simulink library "Ampere_Library"  (R2022b)
settings: Solver=FixedStepDiscrete  StartTime=0  StopTime=10.0  RelTol=1e-3  EnableMultiTasking=on
undefined symbols (not defined in the file or in its folder): A_INST_double, Dem_EventStatusType, ECU_AMBIENT_TEMPERATURE, SET_ECU_AMBIENT_TEMPERATURE, SlDemoSign, Std_ReturnType
libraries: simulink x13
(part 2 of 10)

== system Ampere_Library/User_Defined_Libraries/Discontinuities ==
  note: Saturation and Crossing
  note: Min/Max and DeadZone
  note: Hysteresis and Relays
  note: Discontinuities
  A_DetectSaturation : Subsystem  Tag=[LIB]  mask(A_DetectSaturation){SATOnIntegerOverflow=off}
      mask prompts: SATOnIntegerOverflow "Saturate on integer overflow"
      mask help:
      | Limit input signal to the upper and lower saturation values. Saturation of the [2](input) by entry [1] (maximum) and entry [3] (minimum). Output (sat) will be any of the following values
      |   0 : Input is within the threshold range
      |   1 : Input is less than or equal to minimum threshold
      |   2 : Input is greater than or equal to maximum threshold
      |   3 : The minimum threshold is equal to the maximum threshold.
      |
      | Notes:
      | 1. Second output(sat) is always uint8 datatype.
      | 2. Second output (sat) will be 2
      | if upper saturation value is less than lower saturation value.
      | e.g., if upper is -10 and lower is 10 , then output sat will be 2.
      mask init:
      | %% Internal Parameters
      | SatPas = uint8(0);
      | Satmin = uint8(1);
      | SatMax = uint8(2);
      | UpEqLow = uint8(3);
      settings: AttributesFormatString=%<MaskType>
      mask TypeOptions SATOnIntegerOverflow: Max/SaturateOnIntegerOverflow | Min/SaturateOnIntegerOverflow
      mask Callback SATOnIntegerOverflow:
      | if strcmp(get_param(gcb,'SATOnIntegerOverflow'),'on')
      |     % Display the SaturateOnOverflow parameter
      |     set_param(gcb, 'AttributesFormatString', sprintf('%%<MaskType>\n SAT = on'));
      | else
      |     % Do not display the SaturateOnOverflow parameter
      |     set_param(gcb, 'AttributesFormatString', sprintf('%%<MaskType>\n'));
      | end
      mask Display:
      | %% Plot saturation and axes
      | plot([.8,.6,.4,.2],[.7,.7,.3,.3]);
      | plot([.5,.5],[0.25,.75]);
      | plot([.85,.15],[.5,.5]);
  A_HiThresHys_HighIncl : Subsystem  Tag=[LIB]  mask(A_HiThresHys_HighIncl){Sat_Required=off}
      mask prompts: Sat_Required "Saturate on integer overflow for sum block"
      mask help:
      | Hysteresis Function
      |
      | The block produces a flag that indicates
      | if the input (val) is within the Hysteresis phase
      | defined by hysw (Hysteresis width) and thrs (Threshold).
      |
      | Hys Type  :  Minus
      | Lower Threshold  :  Not Included
      | Upper Threshold  :  Included
      | Lower Hys Flag Value  :  0
      | Upper Hys Flag Value  :  1
      |
      | I/O
      | val     :  Value
      | thrs    :  Threshold Value
      | hysw  :  Hysteresis Width
      |
      | flag :  Answer Flag Value
      |
      | set   : val >= thrs
      | clear : val < thrs - hysw
      | hold  : thrs - hysw <= val < thrs (hold previous value)
      mask init:
      | %% Internal Parameter
      | Initial_condition = 0;
      settings: AttributesFormatString=%<MaskType>
      mask TypeOptions Sat_Required: Sum/SaturateOnIntegerOverflow
      mask Callback Sat_Required:
      | if strcmp(get_param(gcb,'Sat_Required'),'on')
      |     % Display the SaturateOnOverflow parameter
      |     set_param(gcb, 'AttributesFormatString',sprintf('%%<MaskType>\nSAT = on'));
      | else
      |     % Do not display the SaturateOnOverflow parameter
      |     set_param(gcb, 'AttributesFormatString',sprintf('%%<MaskType>\n'));
      | end
      mask Display:
      | %% Data to move up all objects
      | Moveup = .15;
      | 
      | %% Left to right arrow
      | plot([0.62 0.64 0.62], Moveup+[0.27 0.30 0.33]);
      | 
      | %% Right to left arrow
      | plot([0.41 0.39 0.41], Moveup+[0.73 0.70 0.67]);
      | 
      | %% Down up arrow
      | plot([0.62 0.64 0.66], Moveup+[0.66 0.68 0.66]);
      | 
      | %% Up down arrow
      | plot([0.4 0.38 0.36], Moveup+[0.34 0.32 0.34]);
      | 
      | %% Draw paths
      | plot([0.20 0.70], Moveup+[0.30 0.30]);
      | plot([0.64 0.64], Moveup+[0.30 0.70]);
      | plot([0.38 0.80], Moveup+[0.70 0.70]);
      | plot([0.38 0.38], Moveup+[0.30 0.70]);
      | 
      | %% Put texts
      | text(0.60, Moveup+0.15, '   x\n(thrs)');
      | text(0.22, Moveup+0.15, '         z \n(thrs - HysW)');
      | text(0.66, Moveup+0.5, 'val >= x\n   (set)');
      | text(0.41, Moveup+0.5, 'z<=val<x\n  (hold)');
      | text(0.20, Moveup+0.5, 'val < z\n   (clr)');
  A_HiThresHys_LowIncl : Subsystem  Tag=[LIB]  mask(A_HiThresHys_LowIncl){Sat_Required=off}
      mask prompts: Sat_Required "Saturate on integer overflow for Sum Block"
      mask help:
      | Hysteresis Function
      |
      | The block produces a flag that indicates
      | if the input (val) is within the Hysteresis phase
      | defined by hysw (Hysteresis width) and thrs (Threshold).
      |
      | Hys Type  :  Minus
      | Lower Threshold  :  Included
      | Upper Threshold  :  Not Included
      | Lower Hys Flag Value  :  0
      | Upper Hys Flag Value  :  1
      |
      | I/O
      | val     :  Value
      | thrs    :  Threshold Value
      | hysw  :  Hysteresis Width
      |
      | flag :  Answer Flag Value
      |
      | set   : val > thrs
      | clear : val <= thrs - hysw
      | hold  : thrs - hysw < val <= thrs (hold previous value)
      mask init:
      | %% Internal Parameter
      | Initial_condition = 0;
      settings: AttributesFormatString=%<MaskType>
      mask TypeOptions Sat_Required: Sum/SaturateOnIntegerOverflow
      mask Callback Sat_Required:
      | if strcmp(get_param(gcb,'Sat_Required'),'on')
      |     % Display the SaturateOnOverflow parameter
      |     set_param(gcb, 'AttributesFormatString',sprintf('%%<MaskType>\nSAT = on'));
      | else
      |     % Do not display the SaturateOnOverflow parameter
      |     set_param(gcb, 'AttributesFormatString',sprintf('%%<MaskType>\n'));
      | end
      mask Display:
      | %% Data to move up all objects
      | Moveup = .15;
      | 
      | %% Left to right arrow
      | plot([0.62 0.64 0.62], Moveup+[0.27 0.30 0.33]);
      | 
      | %% Right to left arrow
      | plot([0.41 0.39 0.41], Moveup+[0.73 0.70 0.67]);
      | 
      | %% Down up arrow
      | plot([0.62 0.64 0.66], Moveup+[0.66 0.68 0.66]);
      | 
      | %% Up down arrow
      | plot([0.4 0.38 0.36], Moveup+[0.34 0.32 0.34]);
      | 
      | %% Draw paths
      | plot([0.20 0.70], Moveup+[0.30 0.30]);
      | plot([0.64 0.64], Moveup+[0.30 0.70]);
      | plot([0.38 0.80], Moveup+[0.70 0.70]);
      | plot([0.38 0.38], Moveup+[0.30 0.70]);
      | 
      | %% Put texts
      | text(0.60, Moveup+0.15, '   x\n(thrs)');
      | text(0.22, Moveup+0.15, '         z \n(thrs - HysW)');
      | text(0.66, Moveup+0.5, 'val > x\n(set)')
      | text(0.41, Moveup+0.5, 'z<val<=x\n  (hold)')
      | text(0.18, Moveup+0.5, 'val <= z\n   (clr)')
  A_HitCrossing : Subsystem  Tag=[LIB]  mask(A_HitCrossing){offset=50, direction=either, tolerance=double tolerance - eps('double'), user_tol=1, Sat_Required=off}
      mask prompts: offset "Hit crossing offset:"; direction "Hit crossing direction"; tolerance "Tolerance for Offset"; user_tol "User Defined Tolerance"; Sat_Required "Saturate on integer overflow"
      mask help: Detects when the input signal 'U' reaches the Hit crossing offset parameter value in the direction specified by the Hit crossing direction parameter. If the input signal crosses the offset value in the specified direction, the block outputs 1 at the crossing time. If the input signal reaches the offset value in the specified direction and then remains at the offset value, the block outputs 'Out' 1 from the hit time till the time when signal leaves the offset value. If the input signal is constant and equal to the offset value, the block outputs 1 only if the direction is either. For variable-step solvers, Simulink takes a time step before and after the hit crossing time.
      mask init:
      | %% Internal Parameter
      | INI_VAL = 0;
      | 
      | %% Update internal blocks depending of the selected HitCrossing
      | switch direction
      |     case 1
      |         % case rising
      |         set_param([gcb '/VarFrom'],'GotoTag','rise_fall_out');
      |         set_param([gcb '/VarFrom1'],'GotoTag','false');
      |         set_param([gcb '/Var_RO1'],'Operator','>=');
      |         set_param([gcb '/Var_RO2'],'Operator','<');
      |         set_param([gcb '/Var_RO3'],'Operator','>');
      |         set_param([gcb '/Var_RO4'],'Operator','<=');
      |     case 2
      |         % case falling
      |         set_param([gcb '/VarFrom'],'GotoTag','rise_fall_out');
      |         set_param([gcb '/VarFrom1'],'GotoTag','false');
      |         set_param([gcb '/Var_RO1'],'Operator','<=');
      |         set_param([gcb '/Var_RO2'],'Operator','>');
      |         set_param([gcb '/Var_RO3'],'Operator','<');
      |         set_param([gcb '/Var_RO4'],'Operator','>=');
      |     case 3
      |         % case either
      |         set_param([gcb '/VarFrom'],'GotoTag','either');
      |         set_param([gcb '/VarFrom1'],'GotoTag','compare_out');
      | end
      | 
      | %% Compute Tolerance
      | switch tolerance
      |     case 1
      |         tol = eps('double');
      |     case 2
      |         tol = eps('single');
      |     case 3
      |         tol = 0;
      |     case 4
      |         tol = user_tol;
      | end
      | 
      | %% Create the infos to display below the block depending of the Mask Options
      | % Always display MaskType
      | Attrib = '%<MaskType>';
      | % Conditionnally adding Tolerance
      | if strcmp(get_param(gcb,'tolerance'),'User Defined')
      |     Attrib = [Attrib '\nTol = %<user_tol>'];
      | end
      | % Conditionnally adding Sat
      | if strcmp(get_param(gcb,'Sat_Required'),'on')
      |     Attrib = [Attrib '\nSAT = on'];
      | end
      | % Update the display
      | set_param(gcb,'AttributesFormatString',Attrib);
      settings: AttributesFormatString=%<MaskType>
      mask TypeOptions direction: rising | falling | either
      mask TypeOptions tolerance: double tolerance - eps('double') | single tolerance - eps('single') | Absolute Zero | User Defined
      mask Callback tolerance:
      | %% Make visible or not the Tolerance (update 2nd element of MaskVisibilities)
      | MaskVisibilities = get_param(gcb,'MaskVisibilities');
      | if strcmp(get_param(gcb,'tolerance'),'User Defined')
      |     MaskVisibilities{4} = 'on';
      | else
      |     MaskVisibilities{4} = 'off';
      | end
      | set_param(gcb,'MaskVisibilities',MaskVisibilities);
      mask TypeOptions Sat_Required: Add/SaturateOnIntegerOverflow | Add1/SaturateOnIntegerOverflow
      mask Display:
      | %% Plot horizontal and diagonal lines
      | plot([-1,1],[0,0]);
      | plot([-1,1],[-1,1]);
      | 
      | %% Plot the arrows depending of the mask option
      | if strcmp(get_param(gcb,'direction'),'either')
      |     plot([0,0],[-.5,.5]); % centre line
      |     plot([-.1,0],[.3,.5]); % upward arrow
      |     plot([0,.1],[.5,.3]); % upward arrow
      |     plot([0,.1],[-.5,-.3]) % down arrow
      |     plot([0,-.1],[-.5,-.3]) % down arrow
      | elseif strcmp(get_param(gcb,'direction'),'rising')
      |     plot([0,0],[0,.5]); % centre line
      |     plot([-.1,0],[.3,.5]); % upward line
      |     plot([0,.1],[.5,.3]); % upward arrow
      | elseif strcmp(get_param(gcb,'direction'),'falling')
      |     plot([0,0],[0,-.5]); % centre line
      |     plot([0,.1],[-.5,-.3]); % down arrow
      |     plot([0,-.1],[-.5,-.3]); % down arrow
      | end
      | 
      | %% Add the Offset value above as text
      | text(0,.85,sprintf('Offset = %s', get(gcbh,'offset')),'HorizontalAlignment','center')
  A_Hysteresis : Subsystem  Tag=[LIB]  mask(A_Hysteresis){}
      mask help:
      | Aim of this function is to define two ranges for control relay. The Block switches the output from 0 to 1 when the input is greater than or equal to the High, provided High value is greater than the Low.
      | The block switches the output from 1 to 0 when the input is less than or equal to Low value, provided Low value is less than the High.
      |
      | Note: Output Datatype is always "boolean".
      mask init:
      | %% Internal Parameters
      | HysIni = 0;
      settings: AttributesFormatString=%<MaskType>
  A_Hysteresis_Ext_Values : Subsystem  Tag=[LIB]  mask(A_Hysteresis_Ext_Values){Th1_Strict=on, Th2_Strict=on, SaturateOnIntegerOverflow=off}
      mask prompts: Th1_Strict "Output Value 1 when Input falls to Threshold 1"; Th2_Strict "Output Value 2 when Input increases to Threshold 2"; SaturateOnIntegerOverflow "Simulink:blkprm_prompts:AllBlksSaturate"
      mask help:
      | This block outputs 'Value 1' if 'Inp' is lower than 'Threshold 1', and 'Value 2' if 'Inp' is upper than 'Threshold 2'. Between these two values, there is a hysteresis. When both the parameters are cleared, if the input is upper than 'Threshold 2' then the output will be 'Value 2' otherwise it maintains the previous value.
      |
      | Initially, If 'Inp' is in between 'Threshold 1' and 'Threshold 2', then output will be the default value.
      mask init:
      | %% Internal Parameter
      | UDEIC_zero = 0;
      | 
      | %% Parameters used to plot the icon
      | dot_x = [-0.02 -0.014 0 0.014 0.02 0.014 0 -0.014 -0.02];
      | dot_y = [0 0.014 0.02 0.014 0 -0.014 -0.02 -0.014 0];
      | Val1 = 0.2;
      | Val2 = 0.82;
      | Open_T1 = dot_y + Val2;
      | Closed_T1 = dot_y + Val1;
      | Open_T2 = dot_y + Val1;
      | Closed_T2 = dot_y + Val2-0.01;
      | Path_y = [Val1 Val1 Val2 Val2];
      | 
      | %% Update block Th1_Strict and associated icon plot data
      | if Th1_Strict
      |     Th1_falling = 'V1';
      |     Th1_V1 = 1;
      |     Th1_V2 = 0;
      |     set_param([gcb '/RO_Th1Strict'],'Operator','>=');
      |     Open_T1 = dot_y + Val2;
      |     Closed_T1 = dot_y + Val1;
      |     Fall_path_x = [0.2 0.4 0.43 0.8];
      |     Fall_arrow_x = [0.39 0.41 0.43];
      | else
      |     Th1_falling = 'V2';
      |     Th1_V1 = 0;
      |     Th1_V2 = 1;
      |     set_param([gcb '/RO_Th1Strict'],'Operator','>');
      |     Open_T1 = dot_y + Val1;
      |     Closed_T1 = dot_y + Val2-0.01;
      |     Fall_path_x = [0.2 0.37 0.4 0.8];
      |     Fall_arrow_x = [0.36 0.38 0.40];
      | end
      | 
      | %% Update block Th2_Strict and associated icon plot data
      | if Th2_Strict
      |     Th2_rising = 'V2';
      |     Th2_V1 = 0;
      |     Th2_V2 = 1;
      |     set_param([gcb '/RO_Th2Strict'],'Operator','>=');
      |     Open_T2 = dot_y + Val1;
      |     Closed_T2 = dot_y + Val2-0.01;
      |     Rise_path_x = [0.2 0.57 0.6 0.8];
      |     Rise_arrow_x = [0.57 0.59 0.61];
      | else
      |     Th2_rising = 'V1';
      |     Th2_V1 = 1;
      |     Th2_V2 = 0;
      |     set_param([gcb '/RO_Th2Strict'],'Operator','>');
      |     Open_T2 = dot_y + Val2;
      |     Closed_T2 = dot_y + Val1;
      |     Rise_path_x = [0.23 0.6 0.63 0.8];
      |     Rise_arrow_x = [0.6 0.62 0.64];
      | end
      settings: AttributesFormatString=%<MaskType>
      mask TypeOptions SaturateOnIntegerOverflow: Switch/SaturateOnIntegerOverflow | Switch1/SaturateOnIntegerOverflow | SwitchInit/SaturateOnIntegerOverflow
      mask Callback SaturateOnIntegerOverflow:
      | % Display the SaturateOnOverflow parameter only when 'on'
      | if strcmp(get_param(gcb,'SaturateOnIntegerOverflow'),'on')
      |     set_param(gcb,'AttributesFormatString',sprintf('%%<MaskType>\nSAT = on'));
      | else
      |     set_param(gcb,'AttributesFormatString',sprintf('%%<MaskType>\n'));
      | end
      mask DialogControl SaturateOnIntegerOverflow Prompt: Saturate on integer overflow
      mask Display:
      | %% Plot the different elements of the icon
      | plot(Fall_path_x, Path_y, Rise_path_x, Path_y);
      | 
      | plot(Fall_arrow_x, [0.45 0.4 0.45]);
      | plot(Rise_arrow_x, [0.55 0.6 0.55]);
      | 
      | plot(dot_x+0.4, Open_T1);
      | patch(dot_x+0.4, Closed_T1, [0 0 0]);
      | 
      | plot(dot_x+0.6, Open_T2);
      | patch(dot_x+0.6, Closed_T2, [0 0 0]);
      | 
      | %% Put the texts T1/T2/V1/V2
      | disp([repmat(newline,1,2) repmat(' ',1,9) 'T1' repmat(' ',1,6) 'T2' repmat(newline,1,2)]);
      | disp([repmat(newline,1,5) 'v1' repmat(' ',1,27)]);
      | disp([repmat(' ',1,27) 'v2' repmat(newline,1,7)]);
  A_Hysteresis_WithConf : Subsystem  Tag=[LIB]  mask(A_Hysteresis_WithConf){Th1_Strict=on, Th2_Strict=off, int_dt=off, SaturateOnIntegerOverflow=off}
      mask prompts: Th1_Strict "Output Value 1 when Inputfalls to Threshold 1"; Th2_Strict "Output Value 2 when Input increases to Threshold 2"; int_dt "Tick if datatype of Confirmation time is integer with resolution 1"; SaturateOnIntegerOverflow "Simulink:blkprm_prompts:AllBlksSaturate"
      mask help:
      | This block outputs 'Value 1' if 'Inp' is lower than 'Threshold 1' during 'ConfirmationTime', and 'Value 2' if 'Inp' is upper than 'Threshold 2' during 'ConfirmationTime'. Between these two values, there is a hysteresis. If 'Inp' is in between 'Threshold 1' and 'Threshold 2', then previous value will be maintained as output.
      |
      | NOTE: For the first frame, if 'Input' is in between 'Threshold 1' and 'Threshold 2', then default value will be the output
      mask init:
      | %% Parameters used to plot the icon
      | dot_x = [-0.02 -0.014 0 0.014 0.02 0.014 0 -0.014 -0.02];
      | dot_y = [0 0.014 0.02 0.014 0 -0.014 -0.02 -0.014 0];
      | Val1 = 0.2; 
      | Val2 = 0.82;
      | Open_T1 = dot_y + Val2;
      | Closed_T1 = dot_y + Val1;
      | Open_T2 = dot_y + Val1;
      | Closed_T2 = dot_y + Val2-0.01;
      | Path_y = [Val1 Val1 Val2 Val2];
      | 
      | %% Internal Parameters
      | Tim1Ini = 0;
      | Cons_One = 1;
      | Cons_Zero = 0;
      | Boosting_FLP = 1000;
      | Boosting_FXP = 1;
      | timeoutinit = 0;
      | initinit = 0;
      | UDEIC_zero = 0;
      | 
      | %% Update From tags depending of the mask option
      | if strcmp(get_param(gcb,'int_dt'),'on')
      |     set_param([gcb '/ForEachTurnOnDelay/From11'],'GotoTag','Cons_One');
      |     set_param([gcb '/ForEachTurnOnDelay/From13'],'GotoTag','Cons_One');
      | else
      |     set_param([gcb '/ForEachTurnOnDelay/From11'],'GotoTag','tolcons');
      |     set_param([gcb '/ForEachTurnOnDelay/From13'],'GotoTag','tolcons');
      | end
      | 
      | %% Update block Th1_Strict and associated icon plot data
      | if Th1_Strict
      |     Th1_falling = 'V1';
      |     Th1_V1 = 1;
      |     Th1_V2 = 0;
      |     set_param([gcb '/RO_Th1Strict'],'Operator','>=');
      |     Open_T1 = dot_y + Val2;
      |     Closed_T1 = dot_y + Val1;
      |     Fall_path_x = [0.2 0.4 0.43 0.8];
      |     Fall_arrow_x = [0.39 0.41 0.43];
      | else
      |     Th1_falling = 'V2';
      |     Th1_V1 = 0;
      |     Th1_V2 = 1;
      |     set_param([gcb '/RO_Th1Strict'],'Operator','>');
      |     Open_T1 = dot_y + Val1;
      |     Closed_T1 = dot_y + Val2-0.01;
      |     Fall_path_x = [0.2 0.37 0.4 0.8];
      |     Fall_arrow_x = [0.36 0.38 0.40];
      | end
      | 
      | %% Update block Th2_Strict and associated icon plot data
      | if Th2_Strict
      |     Th2_rising = 'V2';
      |     Th2_V1 = 0;
      |     Th2_V2 = 1;
      |      set_param([gcb '/RO_Th2Strict'],'Operator','>=');
      |     Open_T2 = dot_y + Val1;
      |     Closed_T2 = dot_y + Val2-0.01;
      |     Rise_path_x = [0.2 0.57 0.6 0.8];
      |     Rise_arrow_x = [0.57 0.59 0.61];
      | else
      |     Th2_rising = 'V1';
      |     Th2_V1 = 1;
      |     Th2_V2 = 0;
      |     set_param([gcb '/RO_Th2Strict'],'Operator','>');
      |     Open_T2 = dot_y + Val2;
      |     Closed_T2 = dot_y + Val1;
      |     Rise_path_x = [0.23 0.6 0.63 0.8];
      |     Rise_arrow_x = [0.6 0.62 0.64];
      | end
      settings: AttributesFormatString=|
      | %<MaskType>
      | Confirmation Time Integer = %<int_dt>
      mask TypeOptions SaturateOnIntegerOverflow: ForEachTurnOnDelay/DataTypeConversion2/SaturateOnIntegerOverflow | ForEachTurnOnDelay/Product/SaturateOnIntegerOverflow | ForEachTurnOnDelay/Product1/SaturateOnIntegerOverflow | ForEachTurnOnDelay/Subtract4/SaturateOnIntegerOverflow | ForEachTurnOnDelay/Sum/SaturateOnIntegerOverflow | ForEachTurnOnDelay/Switch3/SaturateOnIntegerOverflow | ForEachTurnOnDelay/Switch4/SaturateOnIntegerOverflow | ForEachTurnOnDelay/Switch5/SaturateOnIntegerOverflow | Init/SaturateOnIntegerOverflow | Switch/SaturateOnIntegerOverflow | Switch1/SaturateOnIntegerOverflow
      mask Callback SaturateOnIntegerOverflow:
      | % Display the SaturateOnOverflow parameter only when 'on'
      | if strcmp(get_param(gcb,'SaturateOnIntegerOverflow'),'on')
      |     set_param(gcb,'AttributesFormatString',sprintf('%%<MaskType>\nConfirmation Time Integer = %%<int_dt>\nSAT = on'));
      | else
      |     set_param(gcb,'AttributesFormatString',sprintf('%%<MaskType>\nConfirmation Time Integer = %%<int_dt>'));
      | end
      mask DialogControl SaturateOnIntegerOverflow Prompt: Saturate on integer overflow
      mask Display:
      | %% Plot the different elements of the icon
      | plot(Fall_path_x,Path_y,Rise_path_x,Path_y);
      | 
      | plot(Fall_arrow_x,[0.45 0.4 0.45]);
      | plot(Rise_arrow_x,[0.55 0.6 0.55]);
      | 
      | plot(dot_x+0.4,Open_T1);
      | patch(dot_x+0.4,Closed_T1,[0 0 0]);
      | plot(dot_x+0.35,Open_T1-0.68);
      | plot([dot_x(3),dot_x(5)]+0.35,[Open_T1(3)-0.02,Open_T1(5)]-0.68);
      | plot([dot_x(3),dot_x(3)+(dot_x(4)-dot_x(3))/2]+0.35,[Open_T1(3)-0.02,(Open_T1(3)-0.02)+(Open_T1(4)-Open_T1(3)+0.02)/2]-0.68);
      | 
      | plot(dot_x+0.6,Open_T2);
      | plot(dot_x+0.65,Open_T2+0.05);
      | plot([dot_x(3),dot_x(5)]+0.65,[Open_T1(3)-0.02,Open_T1(5)]+0.05);
      | plot([dot_x(3),dot_x(3)+(dot_x(4)-dot_x(3))/2]+0.65,[Open_T1(3)-0.02,(Open_T1(3)-0.02)+(Open_T1(4)-Open_T1(3)+0.02)/2]+0.05);
      | patch(dot_x+0.6,Closed_T2,[0 0 0]);
      | 
      | %% Put the texts T1/T2/V1/V2
      | disp([repmat(newline,1,2) repmat(' ',1,9) 'T1' repmat(' ',1,6) 'T2' repmat(newline,1,2)]);
      | disp([repmat(newline,1,5) 'v1' repmat(' ',1,27)])
      | disp([repmat(' ',1,27) 'v2' repmat(newline,1,7)]);
  A_LowThresHys_HighIncl : Subsystem  Tag=[LIB]  mask(A_LowThresHys_HighIncl){Sat_Required=off}
      mask prompts: Sat_Required "Saturate on integer overflow for sum block"
      mask help:
      | Hysteresis Function
      |
      | Inputs :
      |     val : Value
      |     thrs : Threshold Value
      |     hysw : Hysteresis Width
      | Output :
      |     flag : Answer Flag Value
      |
      | If : val >= thrs + hysw, the output flag will be set to 1.
      |
      | If : val < thrs, the output flag will be set to 0.
      |
      | If : thrs <= val < thrs + hysw, the output flag maintains its previous
      |                                 value (hysteresis phase)
      |
      | Note:
      | All inputs shall have the same datatype
      | Boolean datatype is not allowed as input
      mask init:
      | %% Internal Parameter
      | Init_Val = 0;
      settings: AttributesFormatString=%<MaskType>
      mask TypeOptions Sat_Required: Sum/SaturateOnIntegerOverflow
      mask Callback Sat_Required:
      | if strcmp(get_param(gcb,'Sat_Required'),'on')
      |     % Display the SaturateOnOverflow parameter
      |     set_param(gcb, 'AttributesFormatString',sprintf('%%<MaskType>\nSAT = on'));
      | else
      |     % Do not display the SaturateOnOverflow parameter
      |     set_param(gcb, 'AttributesFormatString',sprintf('%%<MaskType>\n'));
      | end
      mask DialogControl ParamGroupVar Prompt: Parameters
      mask Display:
      | %% Data to move up all objects
      | Moveup = .15;
      | 
      | %% Left to right arrow
      | plot([0.62 0.64 0.62], Moveup+[0.27 0.30 0.33]);
      | 
      | %% Right to left arrow
      | plot([0.41 0.39 0.41], Moveup+[0.73 0.70 0.67]);
      | 
      | %% Down up arrow
      | plot([0.62 0.64 0.66], Moveup+[0.66 0.68 0.66]);
      | 
      | %% Up down arrow
      | plot([0.40 0.38 0.36], Moveup+[0.34 0.32 0.34]);
      | 
      | %% Draw paths
      | plot([0.20 0.70], Moveup+[0.30 0.30]);
      | plot([0.64 0.64], Moveup+[0.30 0.70]);
      | plot([0.38 0.80], Moveup+[0.70 0.70]);
      | plot([0.38 0.38], Moveup+[0.30 0.70]);
      | 
      | %% Put texts
      | text(0.53, Moveup+0.15, '         y\n(thrs + HysW)')
      | text(0.30, Moveup+0.15, '    x \n(thrs)')
      | text(0.66, Moveup+0.5, 'val >= y\n(set)')
      | text(0.41, Moveup+0.5, 'x<=val<y\n  (hold)')
      | text(0.18, Moveup+0.5, 'val < x\n   (clr)')
  A_LowThresHys_LowIncl : Subsystem  Tag=[LIB]  mask(A_LowThresHys_LowIncl){Sat_Required=off}
      mask prompts: Sat_Required "Saturate on integer overflow for sum block"
      mask help:
      | Hysteresis Function
      |
      | Inputs :
      |     val : Value
      |     thrs : Threshold Value
      |     hysw : Hysteresis Width
      | Output :
      |     flag : Answer Flag Value
      |
      | If : val > thrs + hysw, the output flg_ret will be set to 1.
      |
      | If : val <= thrs, the output flg_ret will be set to 0.
      |
      | If : thrs < val <= thrs + hysw, the output flg_ret maintains its previous
      |                                 value (hysteresis phase)
      |
      | Note:
      | All inputs shall have the same datatype
      | Boolean datatype is not allowed as input
      mask init:
      | %% Internal Parameter
      | flag_init = 0;
      settings: AttributesFormatString=%<MaskType>
      mask TypeOptions Sat_Required: Sum/SaturateOnIntegerOverflow
      mask Callback Sat_Required:
      | if strcmp(get_param(gcb,'Sat_Required'),'on')
      |     % Display the SaturateOnOverflow parameter
      |     set_param(gcb, 'AttributesFormatString',sprintf('%%<MaskType>\nSAT = on'));
      | else
      |     % Do not display the SaturateOnOverflow parameter
      |     set_param(gcb, 'AttributesFormatString',sprintf('%%<MaskType>\n'));
      | end
      mask DialogControl ParamGroupVar Prompt: Parameters
      mask Display:
      | %% Data to move up all objects
      | Moveup = .15;
      | 
      | %% Left to right arrow
      | plot([0.62 0.64 0.62], Moveup+[0.27 0.30 0.33]);
      | 
      | %% Right to left arrow
      | plot([0.41 0.39 0.41], Moveup+[0.73 0.70 0.67]);
      | 
      | %% Down up arrow
      | plot([0.62 0.64 0.66], Moveup+[0.66 0.68 0.66]);
      | 
      | %% Up down arrow
      | plot([0.4 0.38 0.36], Moveup+[0.34 0.32 0.34]);
      | 
      | %% Draw paths
      | plot([0.20 0.70], Moveup+[0.30 0.30]);
      | plot([0.64 0.64], Moveup+[0.30 0.70]);
      | plot([0.38 0.80], Moveup+[0.70 0.70]);
      | plot([0.38 0.38], Moveup+[0.30 0.70]);
      | 
      | %% Put texts
      | text(0.53, Moveup+0.15, '         y\n(thrs + HysW)')
      | text(0.30, Moveup+0.15, '    x \n(thrs)')
      | text(0.66, Moveup+0.5, 'val > y\n(set)')
      | text(0.41, Moveup+0.5, 'x<val<=y\n  (hold)')
      | text(0.18, Moveup+0.5, 'val <= x\n   (clr)')
  A_MaxSaturation : Subsystem  Tag=[LIB]  mask(A_MaxSaturation){Max=2, SATOnIntegerOverflow=off}
      mask prompts: Max "Upper limit"; SATOnIntegerOverflow "Saturate on integer overflow for MinMax"
      mask help: This is an upper saturation block which will limit the Input Signal according to the upper limit value specified in the mask.
      settings: AttributesFormatString=%<MaskType>
      mask TypeOptions SATOnIntegerOverflow: MinMax/SaturateOnIntegerOverflow
      mask Callback SATOnIntegerOverflow:
      | % Display the SaturateOnOverflow parameter only when 'on'
      | if strcmp(get_param(gcb,'SATOnIntegerOverflow'),'on')
      |     set_param(gcb,'AttributesFormatString',sprintf('%%<MaskType>\nSAT = on'));
      | else
      |     set_param(gcb,'AttributesFormatString',sprintf('%%<MaskType>\n'));
      | end
      mask Display:
      | %% Display info on the icon
      | fprintf('Upper Limit:\n%s', get(gcbh,'Max'));
  A_MinSaturation : Subsystem  Tag=[LIB]  mask(A_MinSaturation){Min=2, SaturateOnOverflow=off}
      mask prompts: Min "Lower limit"; SaturateOnOverflow "Saturate on integer overflow"
      mask help: This is a lower saturation block which will limit the Input Signal according to the Lower limit value specified in the mask.
      settings: AttributesFormatString=%<MaskType>
      mask TypeOptions SaturateOnOverflow: MinMax/SaturateOnIntegerOverflow
      mask Callback SaturateOnOverflow:
      | % Display the SaturateOnOverflow parameter only when 'on'
      | if strcmp(get_param(gcb,'SaturateOnOverflow'),'on')
      |     set_param(gcb, 'AttributesFormatString',sprintf('%%<MaskType>\nSAT = on'));
      | else
      |     set_param(gcb, 'AttributesFormatString',sprintf('%%<MaskType>\n'));
      | end
      mask Display:
      | %% Display info on the icon
      | fprintf('Lower Limit:\n%s', get(gcbh,'Min'));
  A_NegativeDecreaseDeadZone : Subsystem  Tag=[LIB]  mask(A_NegativeDecreaseDeadZone){DeadBand=1, SATOnIntegerOverflow=off}
      mask prompts: DeadBand "Dead Zone"; SATOnIntegerOverflow "Saturate on integer overflow"
      mask help:
      | The block freezes a positive input to zero and outputs a negative input based on DeadZone range.
      | Deadzone range is calculated based on the previous input value. Hence the decrease of negative inputs can be filtered with the DeadBand.
      |
      | Notes:
      | 1) DeadBand value should be always positive.
      | 2) MINIMUM possible input value = Datatype MIN + DeadBand.
      mask init:
      | %% Internal Parameter
      | IniVal = 0;
      settings: AttributesFormatString=|
      | %<MaskType>
      | Dead Zone = %<DeadBand>
      mask TypeOptions SATOnIntegerOverflow: MinMax/SaturateOnIntegerOverflow | Switch/SaturateOnIntegerOverflow | Sum/SaturateOnIntegerOverflow
      mask Callback SATOnIntegerOverflow:
      | if strcmp(get_param(gcb,'SATOnIntegerOverflow'),'on')
      |     % Display the SaturateOnOverflow parameter
      |     set_param(gcb, 'AttributesFormatString',sprintf('%%<MaskType>\nDead Zone = %%<DeadBand>\nSAT = on'));
      | else
      |     % Do not display the SaturateOnOverflow parameter
      |     set_param(gcb, 'AttributesFormatString',sprintf('%%<MaskType>\nDead Zone = %%<DeadBand>'));
      | end
  A_PositiveIncreaseDeadZone : Subsystem  Tag=[LIB]  mask(A_PositiveIncreaseDeadZone){DeadBand=1, SATOnIntegerOverflow=off}
      mask prompts: DeadBand "Dead Zone"; SATOnIntegerOverflow "Saturate on integer overflow"
      mask help:
      | The block freezes a negative input to zero and outputs a positive input based on DeadZone range.
      | Deadzone range is calculated based on the previous input value. Hence the increase of positive inputs can be filtered with the DeadBand.
      |
      | Notes:
      | 1) DeadBand value should be always positive.
      | 2) MAXIMUM possible input value = DataType MAX - DeadBand.
      mask init:
      | %% Internal Parameter
      | IniVal = 0;
      settings: AttributesFormatString=|
      | %<MaskType>
      | Dead Zone = %<DeadBand>
      mask TypeOptions SATOnIntegerOverflow: MinMax/SaturateOnIntegerOverflow | Sum/SaturateOnIntegerOverflow | Switch/SaturateOnIntegerOverflow
      mask Callback SATOnIntegerOverflow:
      | if strcmp(get_param(gcb,'SATOnIntegerOverflow'),'on')
      |     % Display the SaturateOnOverflow parameter
      |     set_param(gcb, 'AttributesFormatString',sprintf('%%<MaskType>\nDead Zone = %%<DeadBand>\nSAT = on'));
      | else
      |     % Do not display the SaturateOnOverflow parameter
      |     set_param(gcb, 'AttributesFormatString',sprintf('%%<MaskType>\nDead Zone = %%<DeadBand>'));
      | end
  A_Relay : Subsystem  Tag=[LIB]  mask(A_Relay){}
      mask help:
      | Output is true, if given input "In" is greater than or equal to High Value.
      | Output is false, if given input "In" is less than Low value.
      |
      | Note:
      | This block doesnot work with boolean inputs. whereas Output of this block will have Boolean datatype.
      settings: AttributesFormatString=%<MaskType>
      mask Display:
      | %% Plot normalized (/150) using offset for X/Y axis (+40 / +20)
      | plot((40+[0,20,20,15,20,26,20,20,60,60,65,60,54,60,60,20])/150,...
      |     (20+[20,20,60,70,60,70,60,90,90,70,60,70,60,70,20,20])/150,...
      |     (40+[60,80])/150, (20+[90,90])/150)
  A_RelayInv : Subsystem  Tag=[LIB]  mask(A_RelayInv){OutputWhenON=2.5, OutputWhenOFF=2.5, in_IV=0, SaturateOnIntegerOverflow=off}
      mask prompts: OutputWhenON "Output Threshold High"; OutputWhenOFF "Output Threshold Low"; in_IV "Output Default State"; SaturateOnIntegerOverflow "Simulink:blkprm_prompts:AllBlksSaturate"
      mask help: Output the specified 'on' or 'off' value by comparing the input to the specified thresholds. The on/off state of the relay is not affected by input between the upper and lower limits. If at initialization the input value is between the 2 limits, the block returns the default 'on' or 'off' value.
      mask init:
      | %% Internal Parameters
      | IniVal = 0;
      | Cons0 = 0;
      | Cons1 = 1;
      | Cons2 = 2;
      | 
      | %% Compute temp2
      | temp2 = (2-in_IV);
      | if temp2 < 0
      |     temp2 = 0;
      | end
      settings: AttributesFormatString=%<MaskType>\nOutput Threshold High = %<OutputWhenON>\nOutput Threshold Low = %<OutputWhenOFF>\nOutput Default State = %<in_IV>
      mask TypeOptions SaturateOnIntegerOverflow: Multiport_Switch/SaturateOnIntegerOverflow | Switch/SaturateOnIntegerOverflow | Switch1/SaturateOnIntegerOverflow | Switch2/SaturateOnIntegerOverflow | Switch3/SaturateOnIntegerOverflow | Switch4/SaturateOnIntegerOverflow | Switch5/SaturateOnIntegerOverflow
      mask Callback SaturateOnIntegerOverflow:
      | Attrib = '%<MaskType>\nOutput Threshold High = %<OutputWhenON>\nOutput Threshold Low = %<OutputWhenOFF>\nOutput Default State = %<in_IV>';
      | % Add conditionnally the Saturation display
      | if strcmp(get_param(gcb,'SaturateOnIntegerOverflow'),'on')
      |     Attrib = [Attrib '\nSAT = on'];
      | end
      | set(gcbh,'AttributesFormatString',Attrib);
      mask DialogControl SaturateOnIntegerOverflow Prompt: Saturate on integer overflow
      mask Display:
      | %% Plot the reverse delay
      | plot([.8 .4 .4 .4 .4 .2 .6 .6], [.3 .3 .3 .3 .7 .7 .7 .3]);
